simulink model "LQROptimazition"  (R2020a)
settings: Solver=VariableStepAuto  StartTime=0.0  StopTime=15  RelTol=1e-3
values from neighbouring files (symbols this model uses):
  A = [-0.4555 0.0  0.0438  0.0 ... (first row only)    [Proyecto2.m]
  B = [0.1109;0.0131;0.0;0.7157]    [Proyecto2.m]
  C = [1 0 0 0]    [Proyecto2.m]
  K_lqr = Klqr(1:4)    [Proyecto2.m]
  KI = -K_5(5)    [Proyecto2.m]
  KI_lqr = -Klqr(5)    [Proyecto2.m]
  Kpp = K_5(1:4)    [Proyecto2.m]
libraries: simulink x2
settings Model: Creator=daniel  LastModifiedBy=daniel

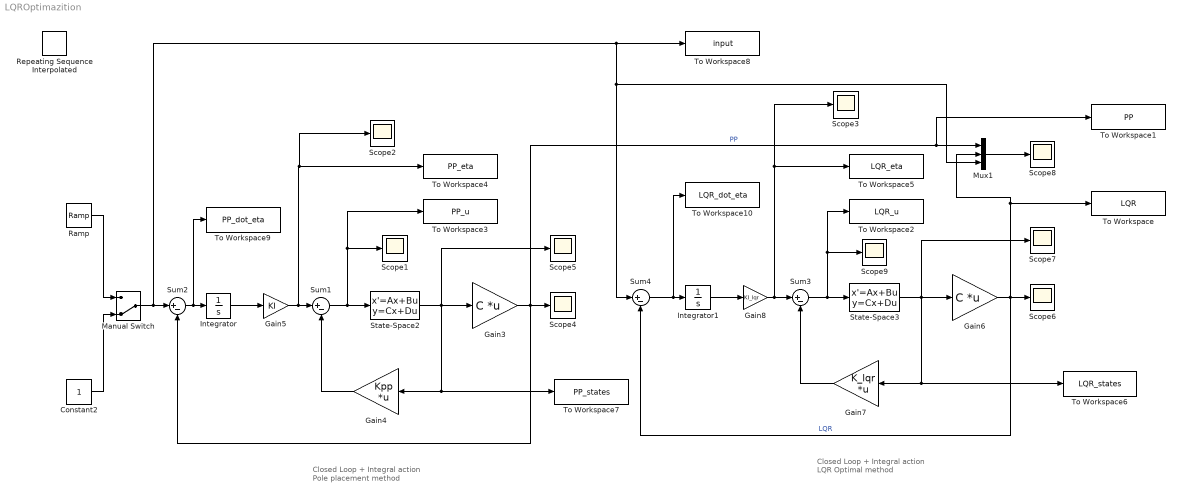
== system LQROptimazition ==
  note: Closed Loop + Integral action
      | Pole placement method
  note: Closed Loop + Integral action
      | LQR Optimal method
  Constant2 : Constant
  Gain3 : Gain  Gain=C  Multiplication=Matrix(K*u) (u vector)
  Gain4 : Gain  Gain=Kpp  Multiplication=Matrix(K*u) (u vector)
  Gain5 : Gain  Gain=KI
  Gain6 : Gain  Gain=C  Multiplication=Matrix(K*u) (u vector)
  Gain7 : Gain  Gain=K_lqr  Multiplication=Matrix(K*u) (u vector)
  Gain8 : Gain  Gain=KI_lqr
  Integrator : Integrator
  Integrator1 : Integrator
  Manual Switch : ManualSwitch  CurrentSetting=0
  Mux1 : Mux  Inputs=3
  Ramp : simulink/Sources/Ramp  slope=1  start=0  InitialOutput=0
  Repeating Sequence Interpolated : simulink/Sources/Repeating Sequence Interpolated  OutValues=[0 1 1 -0.5 -0.5].'  TimeValues=[0 2 10 12 15].'  LookUpMeth=Interpolation-Use End Values  tsamp=0.01  OutMin=[]  OutMax=[]  OutDataTypeStr=double  OutputDataTypeScalingMode=double  OutDataType=fixdt(0,8)  OutScaling=2^-10
  Scope{1..9} (9 alike) : Scope
  State-Space2 : StateSpace  A=A  B=B  C=eye(4)  D=zeros(4,1)  InitialCondition=0
  State-Space3 : StateSpace  A=A  B=B  C=eye(4)  D=zeros(4,1)  InitialCondition=0
  Sum{1..4} (4 alike) : Sum  Inputs=|+-
  To Workspace : ToWorkspace  VariableName=LQR  SampleTime=-1
  To Workspace1 : ToWorkspace  VariableName=PP  SampleTime=-1
      settings: Save2DSignal=2-D array (concatenate along first dimension)
  To Workspace10 : ToWorkspace  VariableName=LQR_dot_eta  SampleTime=-1
      settings: Save2DSignal=2-D array (concatenate along first dimension)
  To Workspace2 : ToWorkspace  VariableName=LQR_u  SampleTime=-1
      settings: Save2DSignal=2-D array (concatenate along first dimension)
  To Workspace3 : ToWorkspace  VariableName=PP_u  SampleTime=-1
      settings: Save2DSignal=2-D array (concatenate along first dimension)
  To Workspace4 : ToWorkspace  VariableName=PP_eta  SampleTime=-1
      settings: Save2DSignal=2-D array (concatenate along first dimension)
  To Workspace5 : ToWorkspace  VariableName=LQR_eta  SampleTime=-1
      settings: Save2DSignal=2-D array (concatenate along first dimension)
  To Workspace6 : ToWorkspace  VariableName=LQR_states  SampleTime=-1
      settings: Save2DSignal=2-D array (concatenate along first dimension)
  To Workspace7 : ToWorkspace  VariableName=PP_states  SampleTime=-1
      settings: Save2DSignal=2-D array (concatenate along first dimension)
  To Workspace8 : ToWorkspace  VariableName=input  SampleTime=-1
      settings: Save2DSignal=2-D array (concatenate along first dimension)
  To Workspace9 : ToWorkspace  VariableName=PP_dot_eta  SampleTime=-1
      settings: Save2DSignal=2-D array (concatenate along first dimension)
  wires:
  Sum1/1 -> Scope1/1, To Workspace3/1, State-Space2/1
  Gain4/1 -> Sum1/2
  Gain3/1 -> To Workspace1/1, Mux1/1, Sum2/2, Scope4/1  "PP"
  State-Space2/1 -> To Workspace7/1, Gain4/1, Scope5/1, Gain3/1
  Gain5/1 -> Scope2/1, To Workspace4/1, Sum1/1
  Integrator/1 -> Gain5/1
  Sum2/1 -> To Workspace9/1, Integrator/1
  State-Space3/1 -> To Workspace6/1, Gain7/1, Scope7/1, Gain6/1
  Integrator1/1 -> Gain8/1
  Sum3/1 -> To Workspace2/1, Scope9/1, State-Space3/1
  Gain6/1 -> To Workspace/1, Mux1/2, Sum4/2, Scope6/1  "LQR"
  Gain7/1 -> Sum3/2
  Sum4/1 -> To Workspace10/1, Integrator1/1
  Gain8/1 -> Scope3/1, To Workspace5/1, Sum3/1
  Mux1/1 -> Scope8/1
  Manual Switch/1 -> Sum4/1, Mux1/3, To Workspace8/1, Sum2/1
  Constant2/1 -> Manual Switch/2
  Ramp/1 -> Manual Switch/1
